simulink model "stateflowlight"  (R2024a)
settings: Solver=FixedStepDiscrete  StartTime=0.0  StopTime=inf  FixedStep=0.1  RelTol=1e-3  EnableMultiTasking=on
settings Model: Creator=hsaiv  LastModifiedBy=hsaiv
settings SolverCC: AlgebraicLoopSolver=TrustRegion  AutoInsertRateTranBlk=on
settings DataIOCC: LimitDataPoints=on
settings OptimizationCC: LifeSpan=inf
settings DebuggingCC: UnconnectedInputMsg=warning  UnconnectedOutputMsg=warning  UnconnectedLineMsg=warning  AllowSymbolicDim=off  SFUnexpectedBacktrackingDiag=warning  SFNoUnconditionalDefaultTransitionDiag=warning  SFExecutionAtInitializationDiag=none  ArithmeticOperatorsInVariantConditions=warning
settings ModelReferenceCC: EnableRefExpFcnMdlSchedulingChecks=on
settings SFSimCC: SimUseLocalCustomCode=off  CustomCodeUndefinedFunction=UseInterfaceOnly
settings RTWCC: RTWUseLocalCustomCode=off  GPUComputeCapability=3.5  DLArmComputeVersion=19.05
settings CodeAppCC: StateflowObjectComments=on
settings GRTTargetCC: TargetLangStandard=C89/C90 (ANSI)
settings ConfigComp: CovMetricSettings=dw  CovSaveCumulativeToWorkspaceVar=on  CovSaveSingleToWorkspaceVar=on  CovExternalEMLEnable=off  CovSFcnEnable=off

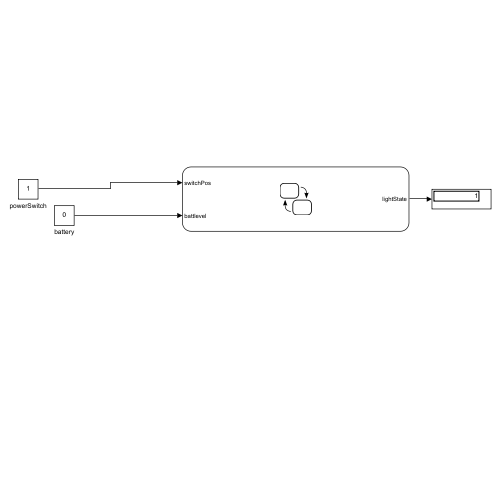
[thumbnail: Simulink's stored preview of the top-level diagram]
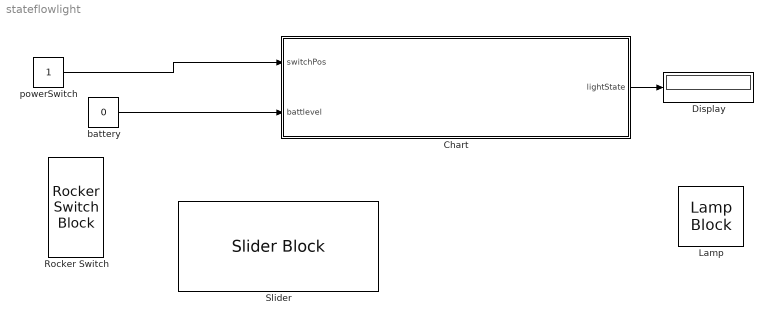
== system stateflowlight ==
  Chart : Stateflow chart  TreatAsAtomicUnit=on
  Display : Display
  Lamp : LampBlock  LabelPosition=Hide
  Rocker Switch : RockerSwitchBlock
      settings: Values={{'Off', 'On'}, [0 1]}
  Slider : SliderBlock
  battery : Constant  Value=0
  powerSwitch : Constant
  wires:
  powerSwitch/1 -> Chart/1(switchPos)
  Chart/1(lightState) -> Display/1
  battery/1 -> Chart/2(battlevel)

== stateflow chart stateflowlight/Chart ==
  state OFF
    entry:
    lightState=0;
  state ON
    entry:
    lightState=1;
  state LOW_BATT
    entry:
    lightState=2;
  (default) -> OFF
  OFF -> ON : [switchPos==1]
  ON -> OFF [order 1] : [switchPos==0]
  (junction 11) -> OFF
  ON -> (junction 14) [order 2] : [battlevel<10]
  (junction 14) -> LOW_BATT
  LOW_BATT -> (junction 11) : after(3,sec)
  data: switchPos input; lightState output; battlevel input
